simulink model "For_Loop_in_Stateflow"  (R2018b)
settings: Solver=FixedStepDiscrete  StartTime=0.0  StopTime=10.0  FixedStep=1  RelTol=1e-3
libraries: simulink x1
settings Model: Creator=marwan  LastModifiedBy=marwan

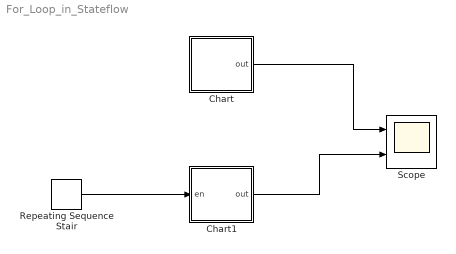
== system For_Loop_in_Stateflow ==
  Chart : Stateflow chart  TreatAsAtomicUnit=on
  Chart1 : Stateflow chart  TreatAsAtomicUnit=on
  Repeating Sequence Stair : simulink/Sources/Repeating Sequence Stair  OutValues=[0 1]  tsamp=-1  OutMin=[]  OutMax=[]  OutDataTypeStr=double  OutputDataTypeScalingMode=double  OutDataType=fixdt(0,8)  ConRadixGroup=Best Precision: Vector-wise  OutScaling=2^-12
  Scope : Scope  NumInputPorts=2
  wires:
  Repeating Sequence Stair/1 -> Chart1/1(en)
  Chart1/1(out) -> Scope/2
  Chart/1(out) -> Scope/1

== stateflow chart For_Loop_in_Stateflow/Chart1 ==
  (default) -> (junction 44)
  (junction 44) -> (junction 45) [order 1] : [en==1]
  (junction 44) -> (junction 46) [order 2] : {out=0}
  (junction 45) -> (junction 56)
  (junction 57) -> (junction 55) [order 1] : [i<=10]
  (junction 55) -> (junction 58) : {out=out+i;}
  (junction 56) -> (junction 57) : {i=1;out=0;}
  (junction 58) -> (junction 57) : {i=i+1;}
  (junction 57) -> (junction 47) [order 2]
  (junction 47) -> (junction 46)
  (junction 46) -> (junction 48)
  data: out output; en input; i local

== stateflow chart For_Loop_in_Stateflow/Chart ==
  (default) -> (junction 9)
  (junction 10) -> (junction 8) [order 1] : [i<=10]
  (junction 8) -> (junction 11) : {out=out+i;}
  (junction 9) -> (junction 10) : {i=1;out=0;}
  (junction 11) -> (junction 10) : {i=i+1;}
  (junction 10) -> (junction 12) [order 2]
  data: out output; i local
